simulink library "Lib_AP_AHRS"  (R2014b)
settings: Solver=ode45  StartTime=0.0  StopTime=10.0  RelTol=1e-3
values from neighbouring files (symbols this model uses):
  kalman_Ak = [1 0 0;0 1 0;0 0 1]    [LoadParameters.m]
  kalman_Hk = [1 0 0;0 1 0;0 0 1]    [LoadParameters.m]
  kalman_p0 = [0 0 0;0 0 0;0 0 0]    [LoadParameters.m]
  kalman_Q = 0.00000001*[1 0 0;0 1 0;0 0 1]    [LoadParameters.m]
  kalman_R = 0.00004*[1 0 0;0 1 0;0 0 1]    [LoadParameters.m]
  kalman_x0 = [0;0;0]    [LoadParameters.m]
libraries: Lib_AP_AHRS x5, simulink x2
settings Model: Creator=Ehang  LastModifiedBy=Ehang

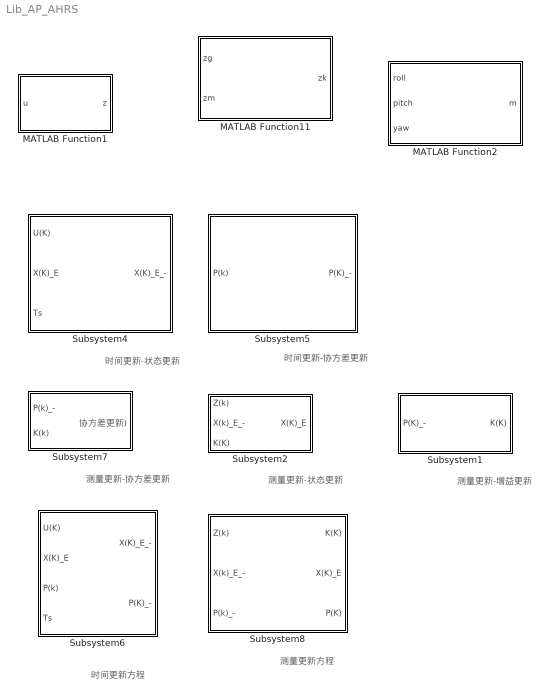
== system Lib_AP_AHRS ==
  note: 测量更新-增益更新
  note: 测量更新-状态更新
  note: 协方差更新
  note: 测量更新-协方差更新
  note: 时间更新方程
  note: 测量更新方程
  note: 时间更新-协方差更新
  note: 时间更新-状态更新
  MATLAB Function1 : MATLAB Function  TreatAsAtomicUnit=on
  MATLAB Function11 : MATLAB Function  TreatAsAtomicUnit=on
  MATLAB Function2 : MATLAB Function  TreatAsAtomicUnit=on
  Subsystem1 : Subsystem
  Subsystem2 : Subsystem
  Subsystem4 : Subsystem
  Subsystem5 : Subsystem
  Subsystem6 : Subsystem
  Subsystem7 : Subsystem
  Subsystem8 : Subsystem

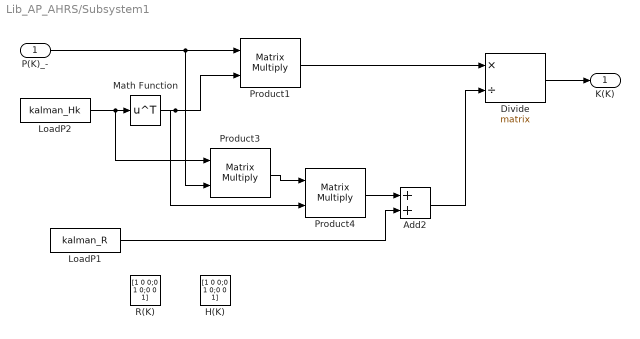
== system Lib_AP_AHRS/Subsystem1 ==
  P(K)_- : Inport
  Add2 : Sum
  Divide : Product  Inputs=*/  Multiplication=Matrix(*)
  H(K) : Constant  Value=[1 0 0;0 1 0;0 0 1]
  LoadP1 : Constant  Value=kalman_R  SampleTime=-1
  LoadP2 : Constant  Value=kalman_Hk  SampleTime=-1
  Math Function : Math  Operator=transpose  SaturateOnIntegerOverflow=on
  Product1 : Product  Multiplication=Matrix(*)  RndMeth=Zero
  Product3 : Product  Multiplication=Matrix(*)  RndMeth=Zero
  Product4 : Product  Multiplication=Matrix(*)  RndMeth=Zero
  R(K) : Constant  Value=[1 0 0;0 1 0;0 0 1]
  K(K) : Outport
  wires:
  LoadP2/1 -> Math Function/1, Product3/1
  Math Function/1 -> Product1/2, Product4/2
  Product1/1 -> Divide/1
  Product3/1 -> Product4/1
  Product4/1 -> Add2/1
  Add2/1 -> Divide/2
  Divide/1 -> K(K)/1
  P(K)_-/1 -> Product1/1, Product3/2
  LoadP1/1 -> Add2/2

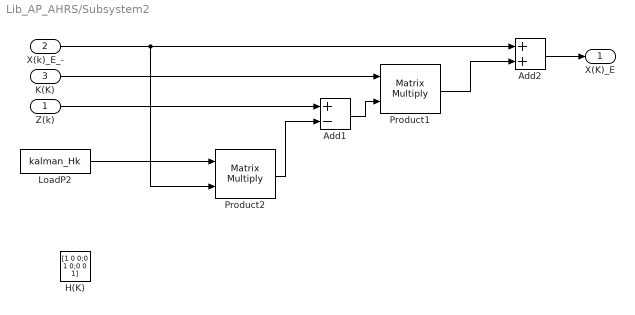
== system Lib_AP_AHRS/Subsystem2 ==
  Z(k) : Inport
  X(k)_E_- : Inport  Port=2
  K(K) : Inport  Port=3
  Add1 : Sum  Inputs=+-
  Add2 : Sum
  H(K) : Constant  Value=[1 0 0;0 1 0;0 0 1]
  LoadP2 : Constant  Value=kalman_Hk  SampleTime=-1
  Product1 : Product  Multiplication=Matrix(*)  RndMeth=Zero
  Product2 : Product  Multiplication=Matrix(*)  RndMeth=Zero
  X(K)_E : Outport
  wires:
  Product2/1 -> Add1/2
  Add1/1 -> Product1/2
  Product1/1 -> Add2/2
  Add2/1 -> X(K)_E/1
  K(K)/1 -> Product1/1
  Z(k)/1 -> Add1/1
  X(k)_E_-/1 -> Product2/2, Add2/1
  LoadP2/1 -> Product2/1

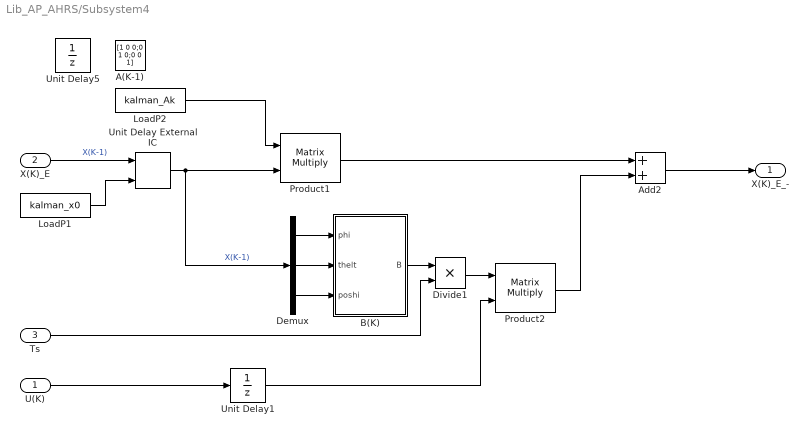
== system Lib_AP_AHRS/Subsystem4 ==
  U(K) : Inport
  X(K)_E : Inport  Port=2
  Ts : Inport  Port=3
  A(K-1) : Constant  Value=[1 0 0;0 1 0;0 0 1]
  Add2 : Sum
  B(K) : Subsystem
  Demux : Demux  Outputs=3
  Divide1 : Product  Inputs=**
  LoadP1 : Constant  Value=kalman_x0  SampleTime=-1
  LoadP2 : Constant  Value=kalman_Ak  SampleTime=-1
  Product1 : Product  Multiplication=Matrix(*)  RndMeth=Zero
  Product2 : Product  Multiplication=Matrix(*)  RndMeth=Zero
  Unit Delay External IC : simulink/Additional Math & Discrete/Additional Discrete/Unit Delay External IC  tsamp=-1
  Unit Delay1 : UnitDelay  InitialCondition=[0;0;0]  SampleTime=-1
  Unit Delay5 : UnitDelay  InitialCondition=[0;0;0]  SampleTime=-1
  X(K)_E_- : Outport
  wires:
  LoadP2/1 -> Product1/1
  Product1/1 -> Add2/1
  Demux/1 -> B(K)/1(phi)
  Demux/2 -> B(K)/2(thelt)
  Demux/3 -> B(K)/3(poshi)
  Unit Delay1/1 -> Product2/2
  Product2/1 -> Add2/2
  Add2/1 -> X(K)_E_-/1
  U(K)/1 -> Unit Delay1/1
  X(K)_E/1 -> Unit Delay External IC/1  "X(K-1)"
  Ts/1 -> Divide1/2
  B(K)/1(B) -> Divide1/1
  Divide1/1 -> Product2/1
  Unit Delay External IC/1 -> Product1/2, Demux/1  "X(K-1)"
  LoadP1/1 -> Unit Delay External IC/2

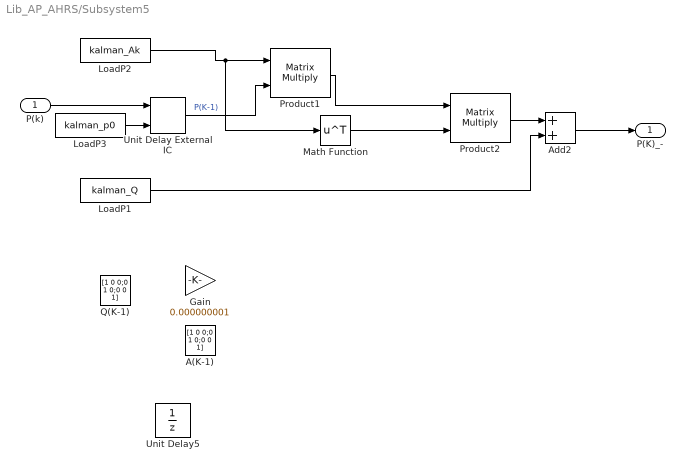
== system Lib_AP_AHRS/Subsystem5 ==
  P(k) : Inport
  A(K-1) : Constant  Value=[1 0 0;0 1 0;0 0 1]
  Add2 : Sum
  Gain : Gain  Gain=0.000000001
  LoadP1 : Constant  Value=kalman_Q  SampleTime=-1
  LoadP2 : Constant  Value=kalman_Ak  SampleTime=-1
  LoadP3 : Constant  Value=kalman_p0  SampleTime=-1
  Math Function : Math  Operator=transpose  SaturateOnIntegerOverflow=on
  Product1 : Product  Multiplication=Matrix(*)  RndMeth=Zero
  Product2 : Product  Multiplication=Matrix(*)  RndMeth=Zero
  Q(K-1) : Constant  Value=[1 0 0;0 1 0;0 0 1]
  Unit Delay External IC : simulink/Additional Math & Discrete/Additional Discrete/Unit Delay External IC  tsamp=-1
  Unit Delay5 : UnitDelay  InitialCondition=[0 0 0;0 0 0;0 0 0]  SampleTime=-1
  P(K)_- : Outport
  wires:
  LoadP2/1 -> Product1/1, Math Function/1
  Unit Delay External IC/1 -> Product1/2  "P(K-1)"
  Product1/1 -> Product2/1
  Math Function/1 -> Product2/2
  Product2/1 -> Add2/1
  LoadP1/1 -> Add2/2
  P(k)/1 -> Unit Delay External IC/1
  Add2/1 -> P(K)_-/1
  LoadP3/1 -> Unit Delay External IC/2

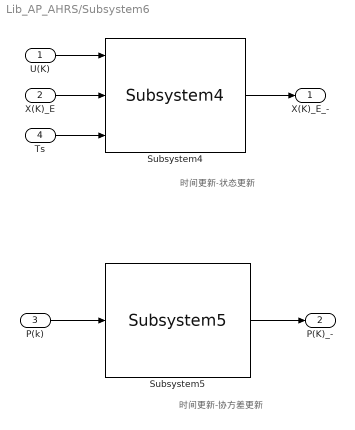
== system Lib_AP_AHRS/Subsystem6 ==
  note: 时间更新-协方差更新
  note: 时间更新-状态更新
  U(K) : Inport
  X(K)_E : Inport  Port=2
  P(k) : Inport  Port=3
  Ts : Inport  Port=4
  Subsystem4 : Lib_AP_AHRS/Subsystem4
  Subsystem5 : Lib_AP_AHRS/Subsystem5
  X(K)_E_- : Outport
  P(K)_- : Outport  Port=2
  wires:
  Subsystem4/1 -> X(K)_E_-/1
  P(k)/1 -> Subsystem5/1
  Subsystem5/1 -> P(K)_-/1
  U(K)/1 -> Subsystem4/1
  X(K)_E/1 -> Subsystem4/2
  Ts/1 -> Subsystem4/3

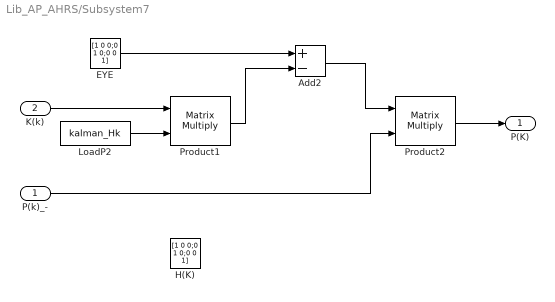
== system Lib_AP_AHRS/Subsystem7 ==
  P(k)_- : Inport
  K(k) : Inport  Port=2
  Add2 : Sum  Inputs=+-
  EYE : Constant  Value=[1 0 0;0 1 0;0 0 1]
  H(K) : Constant  Value=[1 0 0;0 1 0;0 0 1]
  LoadP2 : Constant  Value=kalman_Hk  SampleTime=-1
  Product1 : Product  Multiplication=Matrix(*)  RndMeth=Zero
  Product2 : Product  Multiplication=Matrix(*)  RndMeth=Zero
  P(K) : Outport
  wires:
  EYE/1 -> Add2/1
  Product1/1 -> Add2/2
  Add2/1 -> Product2/1
  Product2/1 -> P(K)/1
  P(k)_-/1 -> Product2/2
  K(k)/1 -> Product1/1
  LoadP2/1 -> Product1/2

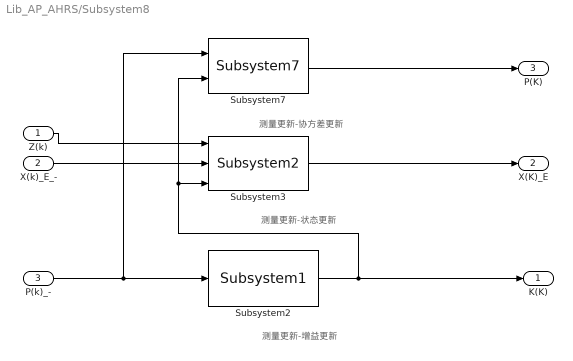
== system Lib_AP_AHRS/Subsystem8 ==
  note: 测量更新-增益更新
  note: 测量更新-状态更新
  note: 测量更新-协方差更新
  Z(k) : Inport
  X(k)_E_- : Inport  Port=2
  P(k)_- : Inport  Port=3
  Subsystem2 : Lib_AP_AHRS/Subsystem1
  Subsystem3 : Lib_AP_AHRS/Subsystem2
  Subsystem7 : Lib_AP_AHRS/Subsystem7
  K(K) : Outport
  X(K)_E : Outport  Port=2
  P(K) : Outport  Port=3
  wires:
  Subsystem2/1 -> K(K)/1, Subsystem3/3, Subsystem7/2
  Subsystem3/1 -> X(K)_E/1
  Subsystem7/1 -> P(K)/1
  Z(k)/1 -> Subsystem3/1
  X(k)_E_-/1 -> Subsystem3/2
  P(k)_-/1 -> Subsystem2/1, Subsystem7/1

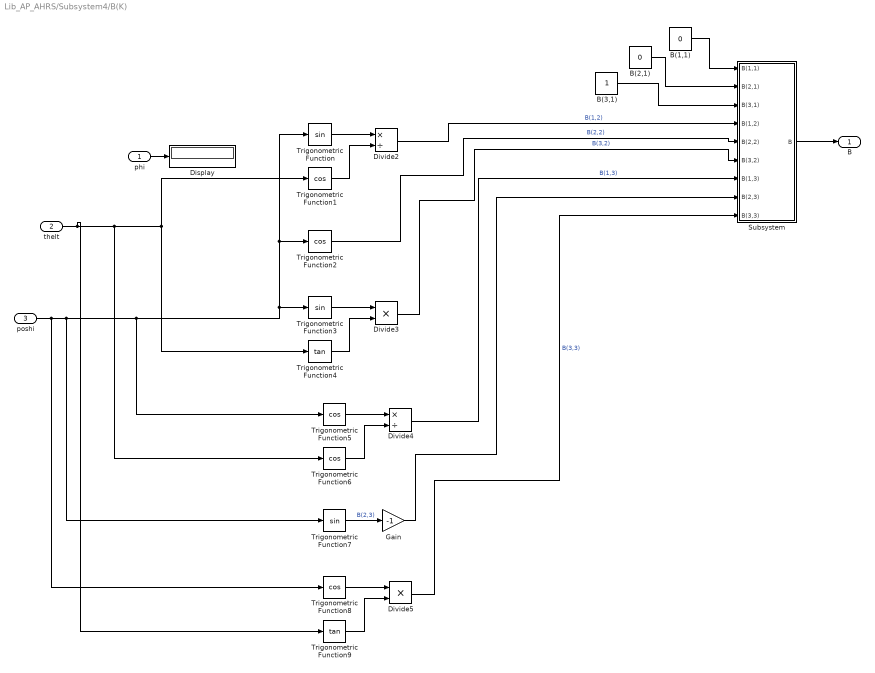
== system Lib_AP_AHRS/Subsystem4/B(K) ==
  phi : Inport
  thelt : Inport  Port=2
  poshi : Inport  Port=3
  B(1,1) : Constant  Value=0  VectorParams1D=off
  B(2,1) : Constant  Value=0  VectorParams1D=off
  B(3,1) : Constant  VectorParams1D=off
  Display : Display
  Divide2 : Product  Inputs=*/
  Divide3 : Product  Inputs=**
  Divide4 : Product  Inputs=*/
  Divide5 : Product  Inputs=**
  Gain : Gain  Gain=-1
  Subsystem : Subsystem
  Trigonometric Function : Trigonometry
  Trigonometric Function{1..2,5..6,8} (5 alike) : Trigonometry  Operator=cos
  Trigonometric Function3 : Trigonometry
  Trigonometric Function4 : Trigonometry  Operator=tan
  Trigonometric Function7 : Trigonometry
  Trigonometric Function9 : Trigonometry  Operator=tan
  B : Outport
  wires:
  Subsystem/1(B) -> B/1
  B(1,1)/1 -> Subsystem/1(B(1,1))
  B(2,1)/1 -> Subsystem/2(B(2,1))
  B(3,1)/1 -> Subsystem/3(B(3,1))
  thelt/1 -> Trigonometric Function9/1, Trigonometric Function6/1, Trigonometric Function4/1, Trigonometric Function1/1
  poshi/1 -> Trigonometric Function8/1, Trigonometric Function7/1, Trigonometric Function5/1, Trigonometric Function3/1, Trigonometric Function2/1, Trigonometric Function/1
  Trigonometric Function/1 -> Divide2/1
  Trigonometric Function1/1 -> Divide2/2
  Divide2/1 -> Subsystem/4(B(1,2))  "B(1,2)"
  Trigonometric Function2/1 -> Subsystem/5(B(2,2))  "B(2,2)"
  Trigonometric Function3/1 -> Divide3/1
  Trigonometric Function4/1 -> Divide3/2
  Divide3/1 -> Subsystem/6(B(3,2))  "B(3,2)"
  Trigonometric Function5/1 -> Divide4/1
  Trigonometric Function6/1 -> Divide4/2
  Divide4/1 -> Subsystem/7(B(1,3))  "B(1,3)"
  Trigonometric Function7/1 -> Gain/1  "B(2,3)"
  Trigonometric Function8/1 -> Divide5/1
  Trigonometric Function9/1 -> Divide5/2
  Divide5/1 -> Subsystem/9(B(3,3))  "B(3,3)"
  Gain/1 -> Subsystem/8(B(2,3))
  phi/1 -> Display/1

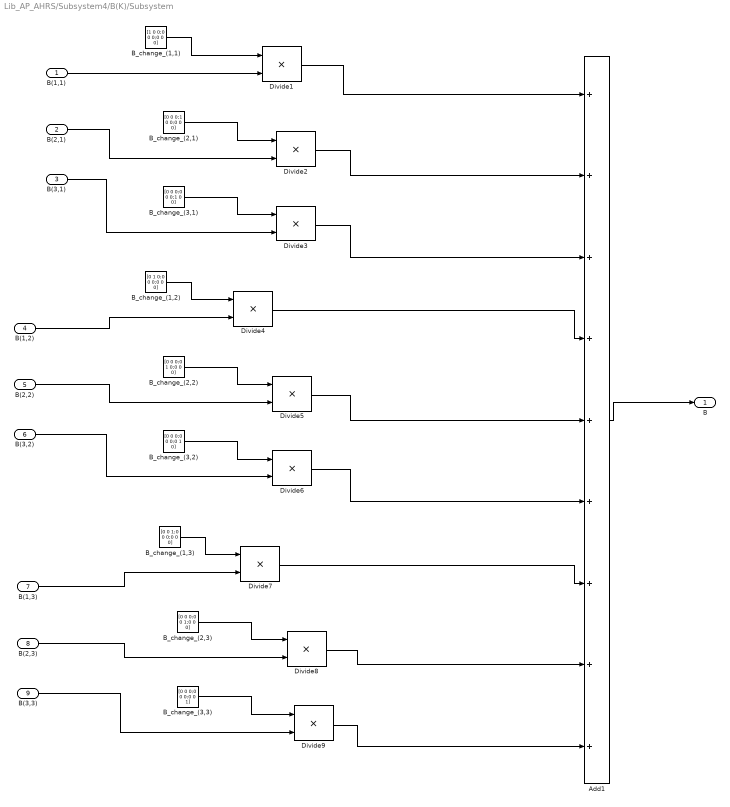
== system Lib_AP_AHRS/Subsystem4/B(K)/Subsystem ==
  B(1,1) : Inport
  B(2,1) : Inport  Port=2
  B(3,1) : Inport  Port=3
  B(1,2) : Inport  Port=4
  B(2,2) : Inport  Port=5
  B(3,2) : Inport  Port=6
  B(1,3) : Inport  Port=7
  B(2,3) : Inport  Port=8
  B(3,3) : Inport  Port=9
  Add1 : Sum  Inputs=+++++++++
  B_change_(1,1) : Constant  Value=[1 0 0;0 0 0;0 0 0]  VectorParams1D=off
  B_change_(1,2) : Constant  Value=[0 1 0;0 0 0;0 0 0]  VectorParams1D=off
  B_change_(1,3) : Constant  Value=[0 0 1;0 0 0;0 0 0]  VectorParams1D=off
  B_change_(2,1) : Constant  Value=[0 0 0;1 0 0;0 0 0]  VectorParams1D=off
  B_change_(2,2) : Constant  Value=[0 0 0;0 1 0;0 0 0]  VectorParams1D=off
  B_change_(2,3) : Constant  Value=[0 0 0;0 0 1;0 0 0]  VectorParams1D=off
  B_change_(3,1) : Constant  Value=[0 0 0;0 0 0;1 0 0]  VectorParams1D=off
  B_change_(3,2) : Constant  Value=[0 0 0;0 0 0;0 1 0]  VectorParams1D=off
  B_change_(3,3) : Constant  Value=[0 0 0;0 0 0;0 0 1]  VectorParams1D=off
  Divide{1..9} (9 alike) : Product  Inputs=**
  B : Outport
  wires:
  B_change_(1,1)/1 -> Divide1/1
  B(1,1)/1 -> Divide1/2
  B_change_(2,1)/1 -> Divide2/1
  B(2,1)/1 -> Divide2/2
  B_change_(3,1)/1 -> Divide3/1
  B(3,1)/1 -> Divide3/2
  B_change_(1,2)/1 -> Divide4/1
  B_change_(2,2)/1 -> Divide5/1
  B_change_(3,2)/1 -> Divide6/1
  B_change_(1,3)/1 -> Divide7/1
  B(1,3)/1 -> Divide7/2
  B_change_(2,3)/1 -> Divide8/1
  B(2,3)/1 -> Divide8/2
  B_change_(3,3)/1 -> Divide9/1
  B(3,3)/1 -> Divide9/2
  Divide1/1 -> Add1/1
  Divide2/1 -> Add1/2
  Divide3/1 -> Add1/3
  Divide4/1 -> Add1/4
  Divide5/1 -> Add1/5
  Divide6/1 -> Add1/6
  Divide7/1 -> Add1/7
  Divide8/1 -> Add1/8
  Divide9/1 -> Add1/9
  B(1,2)/1 -> Divide4/2
  B(2,2)/1 -> Divide5/2
  B(3,2)/1 -> Divide6/2
  Add1/1 -> B/1

== matlab function Lib_AP_AHRS/MATLAB Function11 ==
  data: zg input; zm input; zk output
function zk= monitor(zg,zm)
%#codegen
%% 根据重力加速度求roll和pitch
%pitch 和roll 的计算应该加上0判断的。
pitch=atan(-zg(1)/sqrt(zg(2)*zg(2)+zg(3)*zg(3)));
roll=atan(zg(2)/zg(3));
cr=cos(roll);  sr=sin(roll);
cp=cos(pitch); sp=sin(pitch);

%%根据磁罗盘求yaw，这个自己推到和世科给的结论不一样，要回头重新推到。
%% 橙子推到  检验通过
% yaw=atan((zm(3)*sr-zm(2)*cr)/(zm(1)*cp+zm(2)*sp*sr+zm(3)*sp*cr));
%% 世科推到 检验通过
yaw=atan((-zm(2)*cp+zm(1)*sp*sr)/(zm(1)*cp));
%% 姜推到   检验通过,
% b=(zm(2)*zm(2)+zm(3)*zm(3))/(zm(1)*zm(1)+zm(2)*zm(2)+zm(3)*zm(3));
% temp=(b-sp*sp)/(cp*cp);
% yaw=sign(temp)*asin(sqrt(abs(temp)));%%这一步yaw的值收到了限制，需要改进。
zk=[roll;pitch;yaw];

== matlab function Lib_AP_AHRS/MATLAB Function1 ==
  data: u input; z output
function z=rpy_to_ypr(u)
z=[u(3);u(2);u(1)];

== matlab function Lib_AP_AHRS/MATLAB Function2 ==
  data: roll input; pitch input; m output size=[3,3]; yaw input
function m= to_rotation_matrix(roll,pitch,yaw)
%#codegen
% m=ones(3,3);
cr=cos(roll);  sr=sin(roll);
cp=cos(pitch); sp=sin(pitch);
cy=cos(yaw);   sy=sin(yaw);
% syms cr sr cp sp cy sy
% RZ:Rotate Z axis
% RY:Rotate Y axis
% RX:Rotate X axis
% syms  RZ RY RX
%from earth to body
% RZ:Rotate Z axis
%右旋角度y为正
RZ = [  cy   sy   0;
       -sy   cy   0;
        0    0    1];

% RY:Rotate Y axis
%上仰角度P为正
RY = [  cp   0  -sp;
        0    1    0;
        sp   0   cp];

% RX:Rotate X axis
%右倾角度r为正
RX = [  1    0    0;
        0    cr  sr;
        0   -sr  cr];
%-----------------from_euler-----------------
% column : a b c
% row    : x y z
%                    a                 b      c
% x [            cp*cy,            cp*sy,   -sp]
% y [ cy*sp*sr - cr*sy, cr*cy + sp*sr*sy, cp*sr]
% z [ sr*sy + cr*cy*sp, cr*sp*sy - cy*sr, cp*cr]
% disp('Rotate Matix from earth fixed frame to body fixed frame;');
m= RX*RY*RZ;
% m= [            cp*cy,            cp*sy,   -sp;
%  cy*sp*sr - cr*sy, cr*cy + sp*sr*sy, cp*sr;
% sr*sy + cr*cy*sp, cr*sp*sy - cy*sr, cp*cr];
